simulink model "PE_weightstationary"  (R2022a)
settings: Solver=VariableStepAuto  StartTime=0.0  StopTime=20  RelTol=1e-3
values from neighbouring files (symbols this model uses):
  eta = 0.001    [array_2x2_input.m]
  num_layer = 4    [array_2x2_input.m]
undefined symbols (not defined in the file or in its folder): xc7k70tfbv676
libraries: hdlBasic x77, vmcUtilities x1
(part 2 of 2)

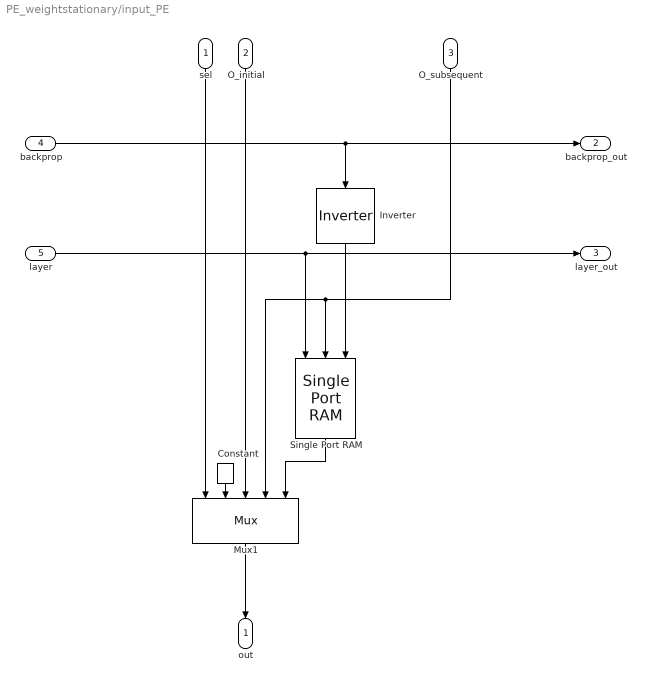
== system PE_weightstationary/input_PE ==
  sel : Inport
  O_initial : Inport  Port=2
  O_subsequent : Inport  Port=3
  backprop : Inport  Port=4
  layer : Inport  Port=5
  Constant : hdlBasic/Constant  const=0  gui_display_data_type=Fixed-point  arith_type=Signed (2's comp)  n_bits=num_bits  bin_pt=frac_bits  preci_type=Single  exp_width=8  frac_width=24  explicit_period=off  period=1  XmcBlockStatus=1  maskContainerNames=tabcontainer1  block_type=constant  block_config=sysgen:Constant_config
  Inverter : hdlBasic/Inverter  en=off  latency=0  XmcBlockStatus=1  maskContainerNames=group2  block_type=inv  block_config=sysgen:Inverter_config
  Mux1 : hdlBasic/Mux  inputs=4  en=off  latency=1  precision=User Defined  arith_type="Signed  (2's comp)"  n_bits=num_bits  bin_pt=frac_bits  quantization=Truncate  overflow=Flag as error  XmcBlockStatus=1  maskContainerNames=tabcontainer1  block_type=mux  block_config=sysgen:Mux_config
  Single Port RAM : hdlBasic/Single Port RAM  depth=num_layer  initVector=zeros(num_layer, 0)  distributed_mem=Block RAM  write_mode=Read After Write  rst=off  init_reg=0  en=off  optimize_latency=off  latency=1  optimize=Area  dbl_ovrd=off  simulation_type=fast_sim  XmcBlockStatus=1  maskContainerNames=tabcontainer1  block_type=spram  block_config=sysgen:SPRAM_config
  out : Outport
  backprop_out : Outport  Port=2
  layer_out : Outport  Port=3
  wires:
  Single Port RAM/1 -> Mux1/5
  O_subsequent/1 -> Single Port RAM/2, Mux1/4
  Constant/1 -> Mux1/2
  layer/1 -> layer_out/1, Single Port RAM/1
  sel/1 -> Mux1/1
  O_initial/1 -> Mux1/3
  Mux1/1 -> out/1
  backprop/1 -> backprop_out/1, Inverter/1
  Inverter/1 -> Single Port RAM/3

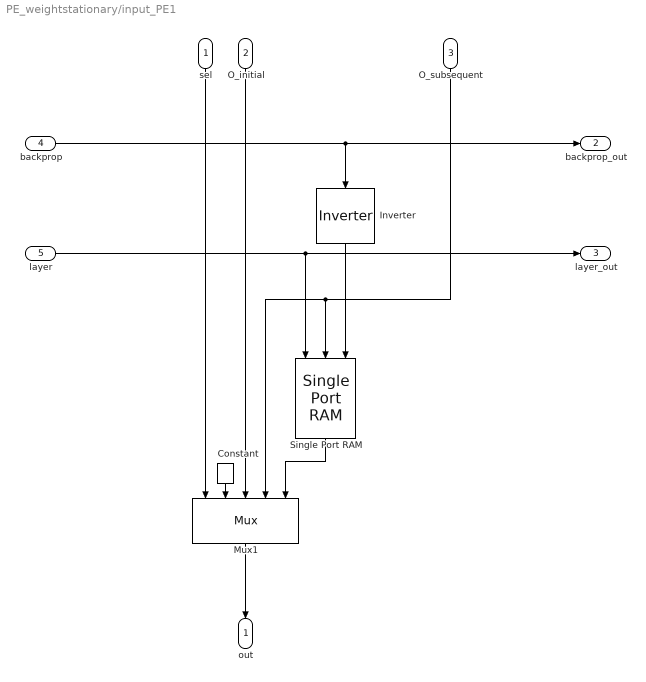
== system PE_weightstationary/input_PE1 ==
  sel : Inport
  O_initial : Inport  Port=2
  O_subsequent : Inport  Port=3
  backprop : Inport  Port=4
  layer : Inport  Port=5
  Constant : hdlBasic/Constant  const=0  gui_display_data_type=Fixed-point  arith_type=Signed (2's comp)  n_bits=num_bits  bin_pt=frac_bits  preci_type=Single  exp_width=8  frac_width=24  explicit_period=off  period=1  XmcBlockStatus=1  maskContainerNames=tabcontainer1  block_type=constant  block_config=sysgen:Constant_config
  Inverter : hdlBasic/Inverter  en=off  latency=0  XmcBlockStatus=1  maskContainerNames=group2  block_type=inv  block_config=sysgen:Inverter_config
  Mux1 : hdlBasic/Mux  inputs=4  en=off  latency=1  precision=User Defined  arith_type="Signed  (2's comp)"  n_bits=num_bits  bin_pt=frac_bits  quantization=Truncate  overflow=Flag as error  XmcBlockStatus=1  maskContainerNames=tabcontainer1  block_type=mux  block_config=sysgen:Mux_config
  Single Port RAM : hdlBasic/Single Port RAM  depth=num_layer  initVector=zeros(num_layer,0)  distributed_mem=Block RAM  write_mode=Read After Write  rst=off  init_reg=0  en=off  optimize_latency=off  latency=1  optimize=Area  dbl_ovrd=off  simulation_type=fast_sim  XmcBlockStatus=1  maskContainerNames=tabcontainer1  block_type=spram  block_config=sysgen:SPRAM_config
  out : Outport
  backprop_out : Outport  Port=2
  layer_out : Outport  Port=3
  wires:
  Single Port RAM/1 -> Mux1/5
  O_subsequent/1 -> Single Port RAM/2, Mux1/4
  Constant/1 -> Mux1/2
  layer/1 -> layer_out/1, Single Port RAM/1
  sel/1 -> Mux1/1
  O_initial/1 -> Mux1/3
  Mux1/1 -> out/1
  backprop/1 -> backprop_out/1, Inverter/1
  Inverter/1 -> Single Port RAM/3
